simulink model "satellite_attitude_kalman_ufk_ekf"  (R2017a)
settings: Solver=FixedStepAuto  StartTime=0.0  StopTime=10.0  FixedStep=dt  RelTol=1e-3
values from neighbouring files (symbols this model uses):
  e = (Ra-Rp)/(Ra+Rp)    [satellite_attitude_kalman_ukf_ekf_run.m]
  i = 45/180*pi    (= 0.785398163397)    [satellite_attitude_kalman_ukf_ekf_run.m]
  qBN_0 = eul2q(InitialEulerO,'xyz','xyzw')    [satellite_attitude_kalman_ukf_ekf_run.m]
  qBO_0 = eul2q(InitialEuler,'xyz','xyzw')    [satellite_attitude_kalman_ukf_ekf_run.m]
  w_BN_0 = [0;2*pi/P;0]    [satellite_attitude_kalman_ukf_ekf_run.m]
  w_ON = [0;2*pi/P;0]    [satellite_attitude_kalman_ukf_ekf_run.m]    (also in satellitekinematics.m = input(4:6,1))
undefined symbols (not defined in the file or in its folder): CONST, Ro, Vo
settings Model: Creator=Rusty Goh  LastModifiedBy=Rusty Goh

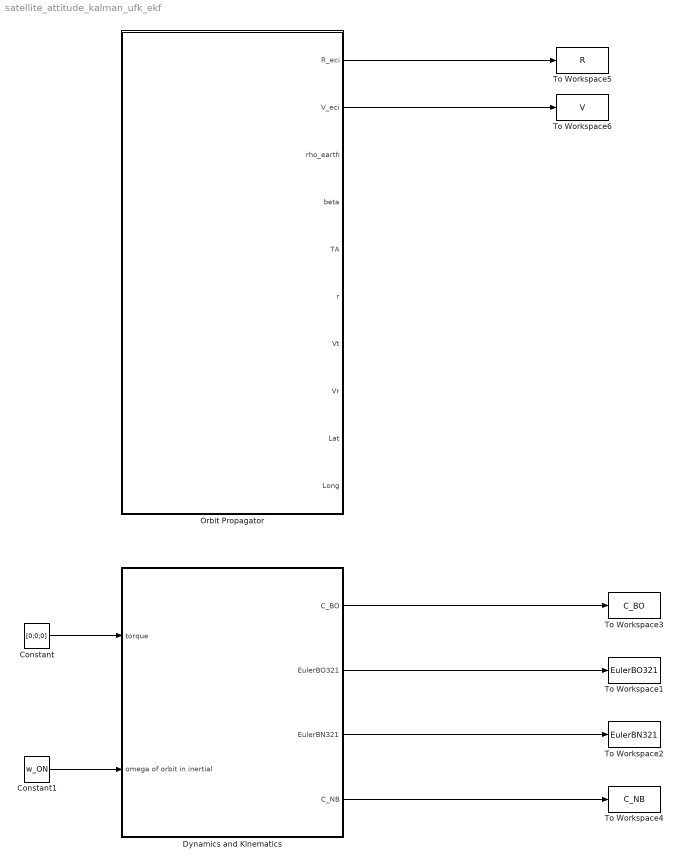
== system satellite_attitude_kalman_ufk_ekf ==
  Constant : Constant  Value=[0;0;0]  VectorParams1D=off
  Constant1 : Constant  Value=w_ON  VectorParams1D=off
  Dynamics and Kinematics : Subsystem
  Orbit Propagator : Subsystem
  To Workspace1 : ToWorkspace  VariableName=EulerBO321  SampleTime=-1
  To Workspace2 : ToWorkspace  VariableName=EulerBN321  SampleTime=-1
  To Workspace3 : ToWorkspace  VariableName=C_BO  SampleTime=-1
  To Workspace4 : ToWorkspace  VariableName=C_NB  SampleTime=-1
  To Workspace5 : ToWorkspace  VariableName=R  SampleTime=-1
  To Workspace6 : ToWorkspace  VariableName=V  SampleTime=-1
  wires:
  Constant/1 -> Dynamics and Kinematics/1(torque)
  Constant1/1 -> Dynamics and Kinematics/2(omega of orbit in inertial)
  Dynamics and Kinematics/1(C_BO) -> To Workspace3/1
  Dynamics and Kinematics/2(EulerBO321) -> To Workspace1/1
  Dynamics and Kinematics/3(EulerBN321) -> To Workspace2/1
  Dynamics and Kinematics/4(C_NB) -> To Workspace4/1
  Orbit Propagator/1(R_eci) -> To Workspace5/1
  Orbit Propagator/2(V_eci) -> To Workspace6/1

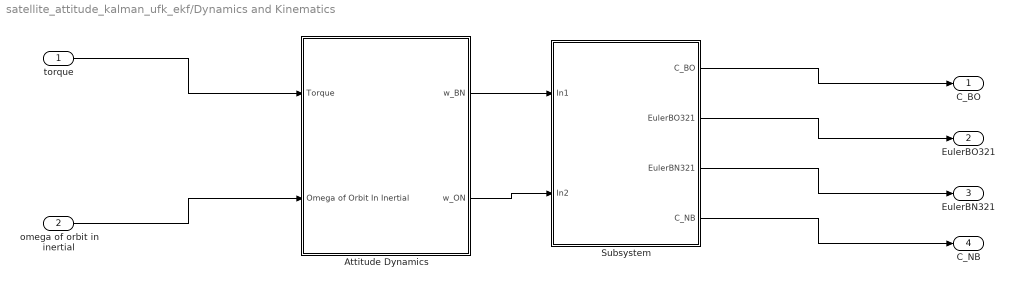
== system satellite_attitude_kalman_ufk_ekf/Dynamics and Kinematics ==
  torque : Inport
  omega of orbit in inertial : Inport  Port=2
  Attitude Dynamics : Subsystem
  Subsystem : Subsystem
  C_BO : Outport
  EulerBO321 : Outport  Port=2
  EulerBN321 : Outport  Port=3
  C_NB : Outport  Port=4
  wires:
  Attitude Dynamics/1(w_BN) -> Subsystem/1(In1)
  Attitude Dynamics/2(w_ON) -> Subsystem/2(In2)
  Subsystem/1(C_BO) -> C_BO/1
  Subsystem/2(EulerBO321) -> EulerBO321/1
  Subsystem/3(EulerBN321) -> EulerBN321/1
  Subsystem/4(C_NB) -> C_NB/1
  torque/1 -> Attitude Dynamics/1(Torque)
  omega of orbit in inertial/1 -> Attitude Dynamics/2(Omega of Orbit In Inertial)

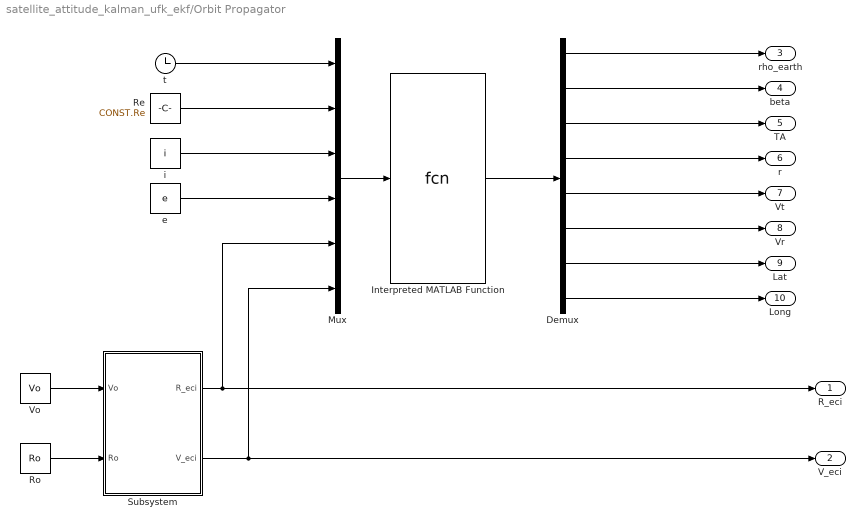
== system satellite_attitude_kalman_ufk_ekf/Orbit Propagator ==
  Demux : Demux  Outputs=8
  Interpreted MATLAB Function : MATLABFcn  MATLABFcn=fcn  OutputDimensions=[8,1]  Output1D=off
  Mux : Mux  Inputs=6
  Re : Constant  Value=CONST.Re
  Ro : Constant  Value=Ro
  Subsystem : Subsystem
  Vo : Constant  Value=Vo
  e : Constant  Value=e
  i : Constant  Value=i
  t : Clock
  R_eci : Outport
  V_eci : Outport  Port=2
  rho_earth : Outport  Port=3
  beta : Outport  Port=4
  TA : Outport  Port=5
  r : Outport  Port=6
  Vt : Outport  Port=7
  Vr : Outport  Port=8
  Lat : Outport  Port=9
  Long : Outport  Port=10
  wires:
  Re/1 -> Mux/2
  e/1 -> Mux/4
  Vo/1 -> Subsystem/1(Vo)
  Subsystem/1(R_eci) -> R_eci/1, Mux/5
  Ro/1 -> Subsystem/2(Ro)
  Subsystem/2(V_eci) -> V_eci/1, Mux/6
  Demux/1 -> rho_earth/1
  Demux/2 -> beta/1
  Demux/3 -> TA/1
  Demux/4 -> r/1
  i/1 -> Mux/3
  Demux/6 -> Vr/1
  Demux/8 -> Long/1
  Demux/5 -> Vt/1
  Interpreted MATLAB Function/1 -> Demux/1
  Demux/7 -> Lat/1
  t/1 -> Mux/1
  Mux/1 -> Interpreted MATLAB Function/1

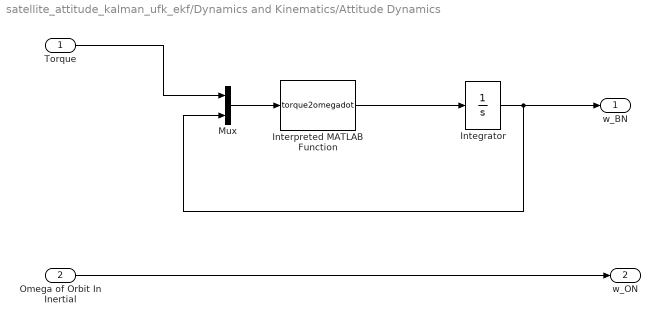
== system satellite_attitude_kalman_ufk_ekf/Dynamics and Kinematics/Attitude Dynamics ==
  Torque : Inport
  Omega of Orbit In Inertial : Inport  Port=2
  Integrator : Integrator  InitialCondition=w_BN_0
  Interpreted MATLAB Function : MATLABFcn  MATLABFcn=torque2omegadot  OutputDimensions=[3,1]  Output1D=off
  Mux : Mux  Inputs=2
  w_BN : Outport
  w_ON : Outport  Port=2
  wires:
  Torque/1 -> Mux/1
  Integrator/1 -> Mux/2, w_BN/1
  Interpreted MATLAB Function/1 -> Integrator/1
  Omega of Orbit In Inertial/1 -> w_ON/1
  Mux/1 -> Interpreted MATLAB Function/1

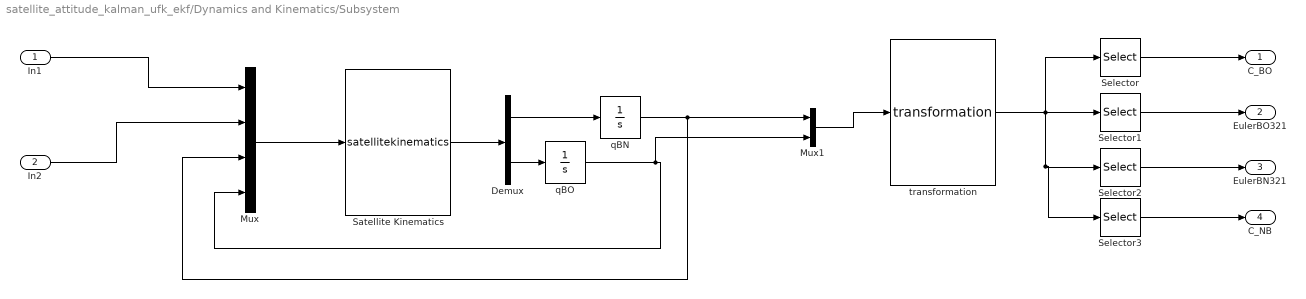
== system satellite_attitude_kalman_ufk_ekf/Dynamics and Kinematics/Subsystem ==
  In1 : Inport
  In2 : Inport  Port=2
  Demux : Demux  Outputs=2
  Mux : Mux
  Mux1 : Mux  Inputs=2
  Satellite Kinematics : MATLABFcn  MATLABFcn=satellitekinematics  OutputDimensions=[8,1]  Output1D=off
  Selector : Selector  NumberOfDimensions=2  InputPortWidth=3  IndexOptions=Index vector (dialog),Index vector (dialog)  Indices=[1:3],[1:3]  OutputSizes=1,1
  Selector1 : Selector  NumberOfDimensions=2  InputPortWidth=3  IndexOptions=Index vector (dialog),Index vector (dialog)  Indices=[1:3],4  OutputSizes=1,1
  Selector2 : Selector  NumberOfDimensions=2  InputPortWidth=3  IndexOptions=Index vector (dialog),Index vector (dialog)  Indices=[1:3],5  OutputSizes=1,1
  Selector3 : Selector  NumberOfDimensions=2  InputPortWidth=3  IndexOptions=Index vector (dialog),Index vector (dialog)  Indices=[1:3],[6:8]  OutputSizes=1,1
  qBN : Integrator  InitialCondition=qBN_0
  qBO : Integrator  InitialCondition=qBO_0
  transformation : MATLABFcn  MATLABFcn=transformation  OutputDimensions=[3,8]  Output1D=off
  C_BO : Outport
  EulerBO321 : Outport  Port=2
  EulerBN321 : Outport  Port=3
  C_NB : Outport  Port=4
  wires:
  In1/1 -> Mux/1
  Mux/1 -> Satellite Kinematics/1
  Mux1/1 -> transformation/1
  In2/1 -> Mux/2
  transformation/1 -> Selector3/1, Selector2/1, Selector1/1, Selector/1
  qBN/1 -> Mux1/1, Mux/3
  Demux/1 -> qBN/1
  Satellite Kinematics/1 -> Demux/1
  Demux/2 -> qBO/1
  qBO/1 -> Mux1/2, Mux/4
  Selector3/1 -> C_NB/1
  Selector1/1 -> EulerBO321/1
  Selector/1 -> C_BO/1
  Selector2/1 -> EulerBN321/1

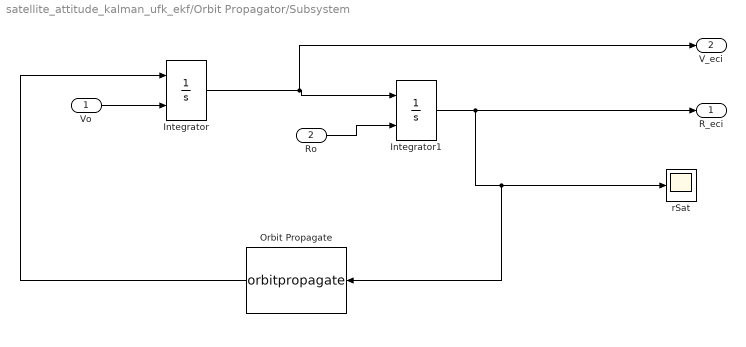
== system satellite_attitude_kalman_ufk_ekf/Orbit Propagator/Subsystem ==
  Vo : Inport
  Ro : Inport  Port=2
  Integrator : Integrator  InitialConditionSource=external
  Integrator1 : Integrator  InitialConditionSource=external
  Orbit Propagate : MATLABFcn  MATLABFcn=orbitpropagate  OutputDimensions=[3,1]  Output1D=off
  rSat : Scope
  R_eci : Outport
  V_eci : Outport  Port=2
  wires:
  Integrator1/1 -> R_eci/1, Orbit Propagate/1, rSat/1
  Vo/1 -> Integrator/2
  Integrator/1 -> V_eci/1, Integrator1/1
  Ro/1 -> Integrator1/2
  Orbit Propagate/1 -> Integrator/1
